simulink model "TLBO_2023"  (R2023b)
settings: Solver=ode45  StartTime=0.0  StopTime=6  MaxStep=1e-4  RelTol=1e-3  EnableMultiTasking=on
PreLoadFcn:
  | Ts_Power=1e-6;
  | Ts_Control=100e-6;
InitFcn:
  | Ts_Power=1e-6;
  | Ts_Control=100e-6;
  | Rtrans=0.142;
  | Xtrans=0.12e-6;
undefined symbols (not defined in the file): DiscIntNeverNeededParam, Ion, Lithium, sigbuilder_block
libraries: dspfdesign x80, spsSeriesRLCBranchLib x52, spsCurrentMeasurementLib x20, spsMeanLib x20, spsIdealSwitchLib x16, spsVoltageMeasurementLib x16, slpidlib x15, spsMosfetLib x14, dspindex x12, spsPWMGeneratorDCDCLib x10, spsGroundLib x10, spsBatteryLib x4
(part 4 of 4)

== system TLBO_2023/Source1/Rooftop Solar System/MPPT ==
  V_PV : Inport
  I_PV : Inport  Port=2
  Add : Sum  Inputs=+-
  Duty Cycle : Constant  Value=Dinit
  MPPT : Subsystem
  PWM Generator (DC-DC) : spsPWMGeneratorDCDCLib/PWM Generator (DC-DC)  Fsw=fc  Ts=Ts_Power
  Saturation : Saturate  UpperLimit=1  LowerLimit=0
  Scope : Scope
  Pulses : Outport  VectorParamsAs1DForOutWhenUnconnected=off
  tag scope: D=global
  wires:
  V_PV/1 -> MPPT/1(V_PV)
  I_PV/1 -> MPPT/2(I_PV)
  PWM Generator (DC-DC)/1 -> Pulses/1
  Saturation/1 -> PWM Generator (DC-DC)/1, [D]
  Add/1 -> Saturation/1, Scope/1  "D"
  MPPT/1(Delta_D) -> Add/2
  Duty Cycle/1 -> Add/1

== system TLBO_2023/Source1/Rooftop Solar System/Pmean ==
  Product : Product  RndMeth=Zero
  WkW : Gain  Gain=1/1000
  P : Outport  VectorParamsAs1DForOutWhenUnconnected=off
  V : Outport  Port=2  VectorParamsAs1DForOutWhenUnconnected=off
  wires:
  [Vmean_PV] -> Product/1, V/1
  Product/1 -> WkW/1
  [Imean_PV] -> Product/2
  WkW/1 -> P/1  "Pmean_PV (kW)"

== system TLBO_2023/Source1/Rooftop Solar System/Subsystem1 ==
  Bus Selector : BusSelector  OutputSignals=V_PV,I_PV,I_diode,Irradiance (W/m2),Temperature (deg C)
  Gain : Gain  Gain=-1
  MPPT Algorithm : Scope
  Mux2 : Mux  Inputs=2
  PV : Scope  NumInputPorts=3
  tag scope: I_PV=global, Idiode_PV=global, Ir=global, Temp=global, V_PV=global
  wires:
  [I_V_MPPT] -> Gain/1  "I_V"
  [V_PV] -> PV/1  "V_PV"
  [I_PV] -> PV/2  "I_PV"
  [Idiode_PV] -> PV/3  "Idiode_PV"
  [dI_dV_MPPT] -> Mux2/1  "dI/dV"
  Gain/1 -> Mux2/2  "-I/V"
  Mux2/1 -> MPPT Algorithm/1  "dI/dV     -I/V (magenta)"
  [m_PV] -> Bus Selector/1
  Bus Selector/1 -> [V_PV]  "<V_PV>"
  Bus Selector/2 -> [I_PV]  "<I_PV>"
  Bus Selector/4 -> [Ir]  "<Irradiance (W/m2)>"
  Bus Selector/3 -> [Idiode_PV]  "<I_diode>"
  Bus Selector/5 -> [Temp]  "<Temperature (deg C)>"

== system TLBO_2023/Source2/Rooftop Solar System/Irradiance Temp ==
  Demux : Demux  Tag=STV Demux  Outputs=2
      settings: DisplayOption=none
  FromWs : FromWorkspace  Tag=STV FromWs  VariableName=tuvar
      SigBuilderData=|
      | common.afterFinalStr = 'Extrapolate'
      | common.sampleTime = '0'
      | dataSet(1).timeRange = [0 1]
      | dataSet(1).name = 'Constant Irradiance'
      | dataSet(2).timeRange = [0 1]
      | dataSet(2).name = 'Step Irradiance'
      | dataSet(3).timeRange = [0 6]
      | dataSet(3).name = 'Ramp-up/down Irradiance'
      | sbobj.Groups(1).Name = 'Constant Irradiance'
      | sbobj.Groups(1).Signals(1).Name = 'Ir'
      | sbobj.Groups(1).Signals(1).XData = [0 1]
      | sbobj.Groups(1).Signals(1).YData = [1000 1000]
      | sbobj.Groups(1).Signals(2).Name = 'Temp'
      | sbobj.Groups(1).Signals(2).XData = [0 1 1 2]
      | sbobj.Groups(1).Signals(2).YData = [0 0 1 1]
      | sbobj.Groups(1).TimeRange = [0 1]
      | sbobj.Groups(2).Name = 'Step Irradiance'
      | sbobj.Groups(2).Signals(1).Name = 'Ir'
      | sbobj.Groups(2).Signals(1).XData = [0 0.252 0.252 1]
      | sbobj.Groups(2).Signals(1).YData = [600 600 1000 1000]
      | sbobj.Groups(2).Signals(2).Name = 'Temp'
      | sbobj.Groups(2).Signals(2).XData = [0 1 1 2]
      | sbobj.Groups(2).Signals(2).YData = [0 0 1 1]
      | sbobj.Groups(2).TimeRange = [0 1]
      | sbobj.Groups(3).Name = 'Ramp-up/down Irradiance'
      | sbobj.Groups(3).Signals(1).Name = 'Ir'
      | sbobj.Groups(3).Signals(1).XData = [0 0.6 1.1 2.2 2.7 6]
      | sbobj.Groups(3).Signals(1).YData = [1000 1000 250 250 1000 1000]
      | sbobj.Groups(3).Signals(2).Name = 'Temp'
      | sbobj.Groups(3).Signals(2).XData = [0 1.5 2.2 3 3.7 6]
      | sbobj.Groups(3).Signals(2).YData = [25 25 28 28 25 25]
      | sbobj.Groups(3).TimeRange = [0 6]
  Ir : Outport  Tag=STV Outport  VectorParamsAs1DForOutWhenUnconnected=off
  Temp : Outport  Tag=STV Outport  Port=2  VectorParamsAs1DForOutWhenUnconnected=off
  wires:
  Demux/1 -> Ir/1
  FromWs/1 -> Demux/1
  Demux/2 -> Temp/1

== system TLBO_2023/Source2/Rooftop Solar System/MPPT ==
  V_PV2 : Inport
  I_PV2 : Inport  Port=2
  Add : Sum  Inputs=+-
  Duty Cycle : Constant  Value=Dinit
  MPPT : Subsystem
  PWM Generator (DC-DC) : spsPWMGeneratorDCDCLib/PWM Generator (DC-DC)  Fsw=fc  Ts=Ts_Power
  Saturation : Saturate  UpperLimit=1  LowerLimit=0
  Scope : Scope
  Pulses : Outport  VectorParamsAs1DForOutWhenUnconnected=off
  tag scope: D2=global
  wires:
  V_PV2/1 -> MPPT/1(V_PV2)
  I_PV2/1 -> MPPT/2(I_PV2)
  PWM Generator (DC-DC)/1 -> Pulses/1
  Saturation/1 -> PWM Generator (DC-DC)/1, [D2]
  Add/1 -> Saturation/1, Scope/1  "D"
  MPPT/1(Delta_D) -> Add/2
  Duty Cycle/1 -> Add/1

== system TLBO_2023/Source2/Rooftop Solar System/Pmean ==
  Product : Product  RndMeth=Zero
  WkW : Gain  Gain=1/1000
  P : Outport  VectorParamsAs1DForOutWhenUnconnected=off
  V : Outport  Port=2  VectorParamsAs1DForOutWhenUnconnected=off
  wires:
  [Vmean_PV2] -> Product/1, V/1
  Product/1 -> WkW/1
  [Imean_PV2] -> Product/2
  WkW/1 -> P/1  "Pmean_PV (kW)"

== system TLBO_2023/Source2/Rooftop Solar System/Subsystem1 ==
  Bus Selector : BusSelector  OutputSignals=V_PV,I_PV,I_diode,Irradiance (W/m2),Temperature (deg C)
  Gain : Gain  Gain=-1
  MPPT Algorithm : Scope
  Mux2 : Mux  Inputs=2
  PV : Scope  NumInputPorts=3
  tag scope: I_PV2=global, Idiode_PV2=global, Ir2=global, Temp2=global, V_PV2=global
  wires:
  [I_V_MPPT2] -> Gain/1  "I_V"
  [V_PV2] -> PV/1  "V_PV"
  [I_PV2] -> PV/2  "I_PV"
  [Idiode_PV2] -> PV/3  "Idiode_PV"
  [dI_dV_MPPT2] -> Mux2/1  "dI/dV"
  Gain/1 -> Mux2/2  "-I/V"
  Mux2/1 -> MPPT Algorithm/1  "dI/dV     -I/V (magenta)"
  [m_PV2] -> Bus Selector/1
  Bus Selector/1 -> [V_PV2]  "<V_PV>"
  Bus Selector/2 -> [I_PV2]  "<I_PV>"
  Bus Selector/4 -> [Ir2]  "<Irradiance (W/m2)>"
  Bus Selector/3 -> [Idiode_PV2]  "<I_diode>"
  Bus Selector/5 -> [Temp2]  "<Temperature (deg C)>"

== system TLBO_2023/Source1/Rooftop Solar System/MPPT/MPPT ==
  note: Maximum power point tracking by incremental conductance method
      | --------------------------------------------------------------
      | Maximum power point is obtained when dP/dV=0  where P= V*I
      | -> d(V*I)/dV = I + V*dI/dV = 0
      | -> dI/dV = -I/V
      |
      | dI, dV  = fundamental components of I and V ripples measured with a sliding time window T_MPPT
      | I , V   = mean values of V and I measured with a sliding time window T_MPPT
      |
      | The integral regulator minimizes the error (dI/dV + I/V)
      | Regulator output = Duty cycle correction
  V_PV : Inport
  I_PV : Inport  Port=2
  Add : Sum  Inputs=+-
  Add1 : Sum
  Dead Zone : DeadZone  LowerValue=-0.05  UpperValue=0.05
  Discrete-Time Integrator : DiscreteIntegrator  SampleTime=Ts_Control  LimitOutput=on  UpperSaturationLimit=1  LowerSaturationLimit=-1  ICPrevOutput=DiscIntNeverNeededParam  ICPrevScaledInput=DiscIntNeverNeededParam
  Fourier : spsFourierLib/Fourier  Freq=1/T_MPPT  n=1  InInit=[0, 0]  Ts=Ts_Control
  Fourier1 : spsFourierLib/Fourier  Freq=1/T_MPPT  n=1  InInit=[0, 0]  Ts=Ts_Control
  MPPT Gain : Gain  Gain=5
  Mean : spsMeanLib/Mean  Freq=1/T_MPPT  Vinit=0  Ts=Ts_Control
  Mean1 : spsMeanLib/Mean  Freq=1/T_MPPT  Vinit=0  Ts=Ts_Control
  Saturation : Saturate  UpperLimit=inf  LowerLimit=eps
  Saturation1 : Saturate  UpperLimit=inf  LowerLimit=eps
  Trigonometric Function : Trigonometry  Operator=cos
  deg2rad : Gain  Gain=pi/180
  div : Product  Inputs=*/  RndMeth=Zero
  div1 : Product  Inputs=**  RndMeth=Zero
  div2 : Product  Inputs=*/  RndMeth=Zero
  Delta_D : Outport  VectorParamsAs1DForOutWhenUnconnected=off
  tag scope: I_V_MPPT=global, Imean_PV=global, Vmean_PV=global, dI_dV_MPPT=global
  wires:
  Dead Zone/1 -> MPPT Gain/1
  Saturation1/1 -> div/2
  Saturation/1 -> div2/2
  Discrete-Time Integrator/1 -> Delta_D/1
  MPPT Gain/1 -> Discrete-Time Integrator/1
  Add1/1 -> Dead Zone/1
  div2/1 -> Add1/2, [I_V_MPPT]  "I/V"
  Mean1/1 -> Saturation/1, [Vmean_PV]
  Mean/1 -> div2/1, [Imean_PV]
  div1/1 -> Add1/1, [dI_dV_MPPT]  "dI/dV"
  Trigonometric Function/1 -> div1/2
  div/1 -> div1/1
  deg2rad/1 -> Trigonometric Function/1
  Add/1 -> deg2rad/1
  Fourier1/1 -> Saturation1/1
  Fourier1/2 -> Add/2
  Fourier/2 -> Add/1
  V_PV/1 -> Mean1/1, Fourier1/1
  I_PV/1 -> Mean/1, Fourier/1
  Fourier/1 -> div/1

== system TLBO_2023/Source2/Rooftop Solar System/MPPT/MPPT ==
  note: Maximum power point tracking by incremental conductance method
      | --------------------------------------------------------------
      | Maximum power point is obtained when dP/dV=0  where P= V*I
      | -> d(V*I)/dV = I + V*dI/dV = 0
      | -> dI/dV = -I/V
      |
      | dI, dV  = fundamental components of I and V ripples measured with a sliding time window T_MPPT
      | I , V   = mean values of V and I measured with a sliding time window T_MPPT
      |
      | The integral regulator minimizes the error (dI/dV + I/V)
      | Regulator output = Duty cycle correction
  V_PV2 : Inport
  I_PV2 : Inport  Port=2
  Add : Sum  Inputs=+-
  Add1 : Sum
  Dead Zone : DeadZone  LowerValue=-0.05  UpperValue=0.05
  Discrete-Time Integrator : DiscreteIntegrator  SampleTime=Ts_Control  LimitOutput=on  UpperSaturationLimit=1  LowerSaturationLimit=-1  ICPrevOutput=DiscIntNeverNeededParam  ICPrevScaledInput=DiscIntNeverNeededParam
  Fourier : spsFourierLib/Fourier  Freq=1/T_MPPT  n=1  InInit=[0, 0]  Ts=Ts_Control
  Fourier1 : spsFourierLib/Fourier  Freq=1/T_MPPT  n=1  InInit=[0, 0]  Ts=Ts_Control
  MPPT Gain : Gain  Gain=5
  Mean : spsMeanLib/Mean  Freq=1/T_MPPT  Vinit=0  Ts=Ts_Control
  Mean1 : spsMeanLib/Mean  Freq=1/T_MPPT  Vinit=0  Ts=Ts_Control
  Saturation : Saturate  UpperLimit=inf  LowerLimit=eps
  Saturation1 : Saturate  UpperLimit=inf  LowerLimit=eps
  Trigonometric Function : Trigonometry  Operator=cos
  deg2rad : Gain  Gain=pi/180
  div : Product  Inputs=*/  RndMeth=Zero
  div1 : Product  Inputs=**  RndMeth=Zero
  div2 : Product  Inputs=*/  RndMeth=Zero
  Delta_D : Outport  VectorParamsAs1DForOutWhenUnconnected=off
  tag scope: I_V_MPPT2=global, Imean_PV2=global, Vmean_PV2=global, dI_dV_MPPT2=global
  wires:
  Dead Zone/1 -> MPPT Gain/1
  Saturation1/1 -> div/2
  Saturation/1 -> div2/2
  Discrete-Time Integrator/1 -> Delta_D/1
  MPPT Gain/1 -> Discrete-Time Integrator/1
  Add1/1 -> Dead Zone/1
  div2/1 -> Add1/2, [I_V_MPPT2]  "I/V"
  Mean1/1 -> Saturation/1, [Vmean_PV2]
  Mean/1 -> div2/1, [Imean_PV2]
  div1/1 -> Add1/1, [dI_dV_MPPT2]  "dI/dV"
  Trigonometric Function/1 -> div1/2
  div/1 -> div1/1
  deg2rad/1 -> Trigonometric Function/1
  Add/1 -> deg2rad/1
  Fourier1/1 -> Saturation1/1
  Fourier1/2 -> Add/2
  Fourier/2 -> Add/1
  V_PV2/1 -> Mean1/1, Fourier1/1
  I_PV2/1 -> Mean/1, Fourier/1
  Fourier/1 -> div/1

== matlab function TLBO_2023/Controller4/Local Controller1 ==
  data: ib_vcs input; b_control output; vbus_vcs input; c_control output; vbus_ref input; mode_vcs input; mode_sc_vcs input
function [b_control, c_control]  = fcn(ib_vcs, vbus_vcs, vbus_ref, mode_vcs, mode_sc_vcs)

% LOCAL CONTROLLER OF BATTERY-CAP SYSTEM
% 
% code to produce error signal from measured value of vbus :
% 
% (i)     Vbus > Vbus_ref +- 5% => charge battery to regulate Vbus
% (ii)    Vbus < Vbus_ref =- 5% => discharge battery to regulate Vbus
% 
% switching is controlled by signals to routers to each power switch

% v_tol = 1.05;
% vbus_max = v_tol*vbus;
% vbus_min = v_tol*vbus;

if(mode_sc_vcs==1)                      %charge state
    c_control = 1;
else                                   %discharge/standby state
    c_control = 0;
end
b_control = 1;

== matlab function TLBO_2023/Controller 2/Local Controller ==
  data: b_control output; vbus_pv2 input; vbus_ref input; mode_pv2 input
function b_control   = fcn(vbus_pv2, vbus_ref, mode_pv2)

% LOCAL CONTROLLER OF BATTERY-CAP SYSTEM
% 
% code to produce error signal from measured value of vbus :
% 
% (i)     Vbus > Vbus_ref => charge battery to regulate Vbus
% (ii)    Vbus < Vbus_ref => discharge battery to regulate Vbus
% 
% switching is controlled by signals to routers to each power switch

if(vbus_pv2>vbus_ref)                  %charge state
    b_control = 0;
else                               %discharge/standby state
    b_control = 1;
end

if(mode_pv2 == 1)
    b_control = 1;
end

== matlab function TLBO_2023/Co-operative Control1/MATLAB Function1 ==
  settings: updateMethod=DISCRETE
  data: I_ref_batt output; I_ref_sc output; mode_batt output; mode_sc output; mode_sc_pcs output; vbus_ref output; mode_sc_vcs output; V_bus input; vbus_pcs input; vbus_vcs input; PV_power input; Load_power input; SoC_batt input; SoC_sc input
function [I_ref_batt, I_ref_sc, mode_batt, mode_sc, mode_sc_pcs, vbus_ref, mode_sc_vcs] = ...
    EMS_TLBO_Simplified_Persistent(V_bus, vbus_pcs, vbus_vcs, PV_power, Load_power, SoC_batt, SoC_sc)
% EMS_TLBO_Simplified_Persistent  % TLBO-based simplified EMS with persistent variables for Simulink
%
%   This function returns fixed-size outputs for code generation and uses
%   persistent TLBO population and fitness values so the optimizer "remembers"
%   past population between Simulink steps.
%
%   Outputs (fixed size):
%       I_ref_batt   - 4x1 battery current reference [A]
%       I_ref_sc     - 2x1 supercap current reference [A]
%       mode_batt    - 4x1 battery mode flags (-1 charge, 0 idle, 1 discharge)
%       mode_sc      - 2x1 supercap mode flags (from vcs & pcs)
%       mode_sc_pcs  - scalar (pcs SC enable flag)
%       vbus_ref     - scalar nominal bus voltage (48 V)
%       mode_sc_vcs  - scalar (vcs SC enable flag)
%
%   Inputs:
%       V_bus        - vector of bus voltages (expected length >= 4)
%       vbus_pcs     - scalar: measured PCS-side bus voltage (for SC mode logic)
%       vbus_vcs     - scalar: measured VCS-side bus voltage (for SC mode logic)
%       PV_power     - vector of PV powers (per MPPT/string)
%       Load_power   - vector of load powers (per load)
%       SoC_batt     - vector length 4 (battery SoC per battery)
%       SoC_sc       - vector length 2 (supercap SoC per SC)
%
%   NOTE: This file is written to be robust: it validates sizes and clips
%   values to bounds. It also uses small eps when dividing by voltages.

% --- Fixed output sizes and defaults ---
I_ref_batt = zeros(4,1);
I_ref_sc   = zeros(2,1);
mode_batt  = zeros(4,1);
mode_sc    = zeros(2,1);
mode_sc_pcs = 0;
mode_sc_vcs = 0;
vbus_ref = 48; % Nominal DC bus voltage

% --- Constants ---
V_nom = 48;       % Nominal bus voltage
P_max_batt = 1000; % Max battery power per channel (W)
P_max_sc   = 500;  % Max supercap power per channel (W)
popSize = 15;      % TLBO population size
dim = 6;           % decision vars: [Pb1 Pb2 Pb3 Pb4 Psc1 Psc2]

% Validate inputs and expand to expected sizes when possible
if isempty(V_bus) || numel(V_bus) < 4
    % If V_bus too short, pad with nominal
    V_bus = V_nom * ones(4,1);
else
    V_bus = V_bus(:); % column
end

if isempty(PV_power), PV_power = 0; end
if isempty(Load_power), Load_power = 0; end

% Ensure SoC vectors have expected sizes (pad with mean if needed)
if isempty(SoC_batt) || numel(SoC_batt) < 4
    SoC_batt = repmat(0.5,4,1); % default 50% SoC
else
    SoC_batt = SoC_batt(:); SoC_batt = SoC_batt(1:4);
end
if isempty(SoC_sc) || numel(SoC_sc) < 2
    SoC_sc = repmat(0.5,2,1);
else
    SoC_sc = SoC_sc(:); SoC_sc = SoC_sc(1:2);
end

% --- Persistent population and fitness ---
persistent Pop Fvec initialized
if isempty(initialized) || isempty(Pop) || isempty(Fvec)
    initialized = true;
    rng('shuffle');
    % Initialize population uniformly in [-Pmax, Pmax]
    Pop = zeros(popSize, dim);
    for i = 1:popSize
        Pop(i,1:4) = -P_max_batt + 2*P_max_batt*rand(1,4); % Battery channels
        Pop(i,5:6) = -P_max_sc + 2*P_max_sc*rand(1,2);   % SC channels
    end
    % Initial fitness values
    Fvec = inf(popSize,1);
    for i = 1:popSize
        Fvec(i) = EMS_cost(Pop(i,:), V_bus, PV_power, Load_power, SoC_batt, SoC_sc, V_nom);
    end
end

% --- TLBO single iteration (teacher + learner) ---
% Teacher phase
[~, idx_best] = min(Fvec);
Xbest = Pop(idx_best,:);
meanPop = mean(Pop,1);
TF = randi([1,2]); % teaching factor 1 or 2
for i = 1:popSize
    r = rand(1,dim);
    Xnew = Pop(i,:) + r.*(Xbest - TF*meanPop);
    % Clip to bounds
    Xnew(1:4) = max(-P_max_batt, min(P_max_batt, Xnew(1:4)));
    Xnew(5:6) = max(-P_max_sc, min(P_max_sc, Xnew(5:6)));
    Jnew = EMS_cost(Xnew, V_bus, PV_power, Load_power, SoC_batt, SoC_sc, V_nom);
    if Jnew < Fvec(i)
        Pop(i,:) = Xnew; Fvec(i) = Jnew;
    end
end

% Learner phase
for i = 1:popSize
    j = randi(popSize);
    while j == i
        j = randi(popSize);
    end
    Xi = Pop(i,:); Xj = Pop(j,:);
    if Fvec(i) < Fvec(j)
        Xnew = Xi + rand(1,dim).*(Xi - Xj);
    else
        Xnew = Xi + rand(1,dim).*(Xj - Xi);
    end
    % Clip to bounds
    Xnew(1:4) = max(-P_max_batt, min(P_max_batt, Xnew(1:4)));
    Xnew(5:6) = max(-P_max_sc, min(P_max_sc, Xnew(5:6)));
    Jnew = EMS_cost(Xnew, V_bus, PV_power, Load_power, SoC_batt, SoC_sc, V_nom);
    if Jnew < Fvec(i)
        Pop(i,:) = Xnew; Fvec(i) = Jnew;
    end
end

% --- Extract best solution ---
[~, idx_best] = min(Fvec);
xbest = Pop(idx_best,:);
Pb = xbest(1:4)';   % 4x1 (W)
Psc = xbest(5:6)';   % 2x1 (W)

% --- Convert power to current references (fixed-size) ---
% Add small eps to avoid division by zero
epsV = 1e-3;
I_ref_batt(:) = Pb(:) ./ (V_bus(1:4) + epsV);
% If V_bus has >=4 entries, use elements 3 and 4 for SC nodes, otherwise use 1:2
if numel(V_bus) >= 4
    I_ref_sc(:) = Psc(:) ./ (V_bus(3:4) + epsV);
else
    I_ref_sc(:) = Psc(:) ./ (V_bus(1:2) + epsV);
end

% --- Mode flags (-1=charge, 1=discharge, 0=idle) ---
mode_batt(:) = sign(Pb(:)); mode_batt(Pb==0) = 0;
mode_sc_local = sign(Psc(:)); mode_sc_local(Psc==0) = 0;

% --- SC mode flags based on voltage thresholds ---
if nargin >= 2 && ~isempty(vbus_pcs)
    if vbus_pcs < 46
        mode_sc_pcs = 1;
    else
        mode_sc_pcs = 0;
    end
end
if nargin >= 3 && ~isempty(vbus_vcs)
    if vbus_vcs < 46
        mode_sc_vcs = 1;
    else
        mode_sc_vcs = 0;
    end
end
% Compose final mode_sc (2x1)
mode_sc = [mode_sc_local(1); mode_sc_local(2)];

end % main function

%% -----------------------------
function J = EMS_cost(P, V_bus, PV_power, Load_power, SoC_batt, SoC_sc, V_nom)
% Fitness function: minimize power mismatch + voltage deviation + usage penalties
% Inputs:
%   P - 1x6 vector: [Pb1 Pb2 Pb3 Pb4 Psc1 Psc2]

Pb = P(1:4);
Psc = P(5:6);

% Power mismatch (scalars)
P_total_storage = sum(Pb) + sum(Psc);
P_total_pv = sum(PV_power(:));
P_total_load = sum(Load_power(:));
P_err = abs(P_total_pv - P_total_load - P_total_storage);

% Voltage deviation cost (target ~V_nom)
V_bus_col = V_bus(:)';
V_err_basic = mean((V_bus_col - V_nom).^2);

% Penalty for being outside 46–50 V
lower_limit = 46; upper_limit = 50;
penalty = 0;
for k = 1:numel(V_bus_col)
    if V_bus_col(k) < lower_limit
        penalty = penalty + (lower_limit - V_bus_col(k));
    elseif V_bus_col(k) > upper_limit
        penalty = penalty + (V_bus_col(k) - upper_limit);
    end
end
V_err = V_err_basic + 5 * penalty; % add strong penalty

% SoC variance penalties (encourage balanced SoC)
SoC_err_batt = sum((SoC_batt(:) - mean(SoC_batt(:))).^2);
SoC_err_sc = sum((SoC_sc(:) - mean(SoC_sc(:))).^2);

% SC usage penalty
SC_penalty = sum(abs(Psc));

% Weighted sum (tunable weights)
w1 = 0.5; w2 = 0.7; w3 = 0.2; w4 = 0.05;
J = w1*V_err + w2*P_err + w3*(SoC_err_batt + SoC_err_sc) + w4*SC_penalty;
end

== matlab function TLBO_2023/Co-operative Control2/MATLAB Function1 ==
  settings: updateMethod=DISCRETE
  data: I_ref_batt output; I_ref_sc output; mode_batt output; mode_sc output; mode_sc_pcs output; vbus_ref output; mode_sc_vcs output; V_bus input; vbus_pcs input; vbus_vcs input; PV_power input; Load_power input; SoC_batt input; SoC_sc input
function [I_ref_batt, I_ref_sc, mode_batt, mode_sc, mode_sc_pcs, vbus_ref, mode_sc_vcs] = ...
    EMS_TLBO_Follow12(V_bus, vbus_pcs, vbus_vcs, PV_power, Load_power, SoC_batt, SoC_sc)

%% Fixed-size outputs
I_ref_batt   = zeros(4,1);   % 4x1
I_ref_sc     = zeros(2,1);   % 2x1
mode_batt    = zeros(4,1);   % 4x1
mode_sc      = zeros(2,1);   % 2x1
mode_sc_pcs  = 0;
mode_sc_vcs  = 0;
vbus_ref     = 48 * ones(4,1); % all buses targeted to 48 V

%% Parameters
V_nom        = 48;
P_max_batt   = 1000;
P_max_sc     = 500;
popSize      = 15;
dim          = 6; % [Pb1 Pb2 Pb3 Pb4 Psc3 Psc4]

lower_limit = 47;
upper_limit = 49.5;
crit_thresh = 47;
penalty_gain = 10;

w_voltage = 0.6;
w_power   = 0.8;
w_soc     = 0.2;
w_sc_use  = 0.05;

% weights for each bus (buses 3 and 4 get extra relative weight)
bus_weights = [1.0, 1.0, 1.0, 1.0];
rel_weight  = 2.0; % weight for V3~V1 and V4~V2 matching

%% Persistent TLBO state
persistent Pop Fvec initialized

if isempty(initialized)
    initialized = true;
    Pop = zeros(popSize, dim);
    for ii = 1:popSize
        Pop(ii,1:4) = -P_max_batt + 2*P_max_batt*rand(1,4);
        Pop(ii,5:6) = -P_max_sc + 2*P_max_sc*rand(1,2);
    end
    Fvec = inf(popSize,1);
    for ii=1:popSize
        Fvec(ii) = EMS_cost_follow12(Pop(ii,:), V_bus, PV_power, Load_power, SoC_batt, SoC_sc, ...
                                      V_nom, lower_limit, upper_limit, crit_thresh, bus_weights, rel_weight, penalty_gain, ...
                                      w_voltage, w_power, w_soc, w_sc_use);
    end
end

%% TLBO teacher phase
[~, idx_best] = min(Fvec);
Xbest = Pop(idx_best,:);
meanPop = mean(Pop,1);
TF = randi([1,2]);
for ii = 1:popSize
    r = rand(1,dim);
    Xnew = Pop(ii,:) + r .* ( Xbest - TF .* meanPop );
    Xnew(1:4) = max(-P_max_batt, min(P_max_batt, Xnew(1:4)));
    Xnew(5:6) = max(-P_max_sc,   min(P_max_sc,   Xnew(5:6)));
    Jnew = EMS_cost_follow12(Xnew, V_bus, PV_power, Load_power, SoC_batt, SoC_sc, ...
                              V_nom, lower_limit, upper_limit, crit_thresh, bus_weights, rel_weight, penalty_gain, ...
                              w_voltage, w_power, w_soc, w_sc_use);
    if Jnew < Fvec(ii)
        Pop(ii,:) = Xnew;
        Fvec(ii) = Jnew;
    end
end

%% TLBO learner phase
for ii = 1:popSize
    jj = randi(popSize);
    while jj == ii
        jj = randi(popSize);
    end
    Xi = Pop(ii,:); Xj = Pop(jj,:);
    if Fvec(ii) < Fvec(jj)
        Xnew = Xi + rand(1,dim) .* (Xi - Xj);
    else
        Xnew = Xi + rand(1,dim) .* (Xj - Xi);
    end
    Xnew(1:4) = max(-P_max_batt, min(P_max_batt, Xnew(1:4)));
    Xnew(5:6) = max(-P_max_sc,   min(P_max_sc,   Xnew(5:6)));
    Jnew = EMS_cost_follow12(Xnew, V_bus, PV_power, Load_power, SoC_batt, SoC_sc, ...
                              V_nom, lower_limit, upper_limit, crit_thresh, bus_weights, rel_weight, penalty_gain, ...
                              w_voltage, w_power, w_soc, w_sc_use);
    if Jnew < Fvec(ii)
        Pop(ii,:) = Xnew;
        Fvec(ii) = Jnew;
    end
end

%% Extract best solution
[~, idx_best] = min(Fvec);
xbest = Pop(idx_best,:);
Pb  = xbest(1:4);
Psc = xbest(5:6);

Pb  = max(-P_max_batt, min(P_max_batt, Pb(:)));
Psc = max(-P_max_sc,   min(P_max_sc,   Psc(:)));

% Current references
Vbus_local = V_bus(:) + 1e-6;
I_ref_batt(:) = Pb(:) ./ Vbus_local(:);
I_ref_sc(:)   = Psc(:) ./ Vbus_local(3:4);

mode_batt(:) = sign(Pb(:));
mode_batt(Pb==0) = 0;
mode_sc(:) = sign(Psc(:));
mode_sc(Psc==0) = 0;

% SC activation flags
mode_sc_pcs = double(vbus_pcs < lower_limit);
mode_sc_vcs = double(vbus_vcs < lower_limit);

end

%% --------------------------
function J = EMS_cost_follow12(P, V_bus, PV_power, Load_power, SoC_batt, SoC_sc, ...
                                V_nom, lower_limit, upper_limit, crit_thresh, bus_weights, rel_weight, penalty_gain, ...
                                w_voltage, w_power, w_soc, w_sc_use)
Pb  = P(1:4); Psc = P(5:6);
total_storage = sum(Pb) + sum(Psc);
total_PV = sum(PV_power(:));
P_err = abs(total_PV - sum(Load_power(:)) - total_storage);

% Voltage deviation from nominal
V_err_basic = sum(bus_weights(:) .* (V_bus(:) - V_nom).^2);

% Relative voltage matching: V3~V1, V4~V2
V_rel_pen = rel_weight * ((V_bus(3)-V_bus(1))^2 + (V_bus(4)-V_bus(2))^2);

% Out-of-band penalties
penalty = 0;
for k = 1:4
    vk = V_bus(k);
    if vk < lower_limit
        penalty = penalty + bus_weights(k) * (lower_limit - vk)^2;
    elseif vk > upper_limit
        penalty = penalty + bus_weights(k) * (vk - upper_limit)^2;
    end
end
if any(V_bus(:) < crit_thresh)
    idx = find(V_bus(:) < crit_thresh);
    penalty = penalty + 200 * sum((crit_thresh - V_bus(idx)).^2);
end
V_err = V_err_basic + V_rel_pen + penalty_gain*penalty;

% SoC penalties
SoC_err = sum((SoC_batt(:)-mean(SoC_batt(:))).^2) + sum((SoC_sc(:)-mean(SoC_sc(:))).^2);

% SC usage penalty
SC_penalty = sum(abs(Psc));

J = w_voltage*V_err + w_power*P_err + w_soc*SoC_err + w_sc_use*SC_penalty;
end

== matlab function TLBO_2023/Controller4/Local Controller ==
  data: b_control output; ib_vcs input; soc_b_vcs input; vbus_vcs input; vbus_ref input
function b_control   = fcn(ib_vcs, soc_b_vcs, vbus_vcs, vbus_ref)

% LOCAL CONTROLLER OF BATTERY-CAP SYSTEM
% 
% code to produce error signal from measured value of vbus :
% 
% (i)     Vbus > Vbus_ref => charge battery to regulate Vbus
% (ii)    Vbus < Vbus_ref => discharge battery to regulate Vbus
% 
% switching is controlled by signals to routers to each power switch

if(vbus_vcs>vbus_ref)                  %charge state
    b_control = 0;
else                               %discharge/standby state
    b_control = 1;
end

== matlab function TLBO_2023/Co-operative Control/MATLAB Function1 ==
  settings: updateMethod=DISCRETE
  data: V_bus input; vbus_pcs input; vbus_vcs input; PV_power input; Load_power input; SoC_batt input; SoC_sc input; I_ref_batt output; I_ref_sc output; mode_batt output; mode_sc output; mode_sc_pcs output; vbus_ref output; mode_sc_vcs output
function [I_ref_batt, I_ref_sc, mode_batt, mode_sc, mode_sc_pcs, vbus_ref, mode_sc_vcs] = ...
    EMS_TLBO_Simplified_Persistent(V_bus, vbus_pcs, vbus_vcs, PV_power, Load_power, SoC_batt, SoC_sc)
% TLBO-based simplified EMS with persistent variables for Simulink
% All outputs are fixed-size for code generation

%% Fixed output sizes
I_ref_batt = zeros(4,1);   % 4x1 battery current
I_ref_sc   = zeros(2,1);   % 2x1 supercap current
mode_batt  = zeros(4,1);   % 4x1 battery mode
mode_sc    = zeros(2,1);   % 2x1 SC mode
vbus_ref   = 48;           % Nominal DC bus voltage
mode_sc_pcs = 0;
mode_sc_vcs = 0;

%% Constants
V_nom = 48;                   % Nominal bus voltage for current calculation
P_max_batt = 100;              % Max battery power
P_max_sc   = 50;               % Max supercap power
popSize    = 15;               % TLBO population size
dim        = 6;                % [Pb1 Pb2 Pb3 Pb4 Psc3 Psc4]

%% SC mode flags based on voltage thresholds
if vbus_pcs < 46, mode_sc_pcs = 1; else mode_sc_pcs = 0; end
if vbus_vcs < 46, mode_sc_vcs = 1; else mode_sc_vcs = 0; end

%% Persistent variables
persistent Pop Fvec initialized

if isempty(initialized)
    initialized = true;
    % Initialize population uniformly in [-Pmax, Pmax]
    Pop = zeros(popSize, dim);
    for i = 1:popSize
        Pop(i,1:4) = -P_max_batt + 2*P_max_batt*rand(1,4);  % Battery
        Pop(i,5:6) = -P_max_sc + 2*P_max_sc*rand(1,2);      % SC
    end
    % Initial fitness values
    Fvec = inf(popSize,1);
    for i=1:popSize
        Fvec(i) = EMS_cost(Pop(i,:), V_bus, PV_power, Load_power, SoC_batt, SoC_sc, V_nom);
    end
end

%% TLBO single iteration (teacher + learner)
% Teacher phase
[~, idx_best] = min(Fvec);
Xbest = Pop(idx_best,:);
meanPop = mean(Pop,1);
TF = randi([1,2]);
for i=1:popSize
    r = rand(1,dim);
    Xnew = Pop(i,:) + r.*(Xbest - TF*meanPop);
    % Clip to bounds
    Xnew(1:4) = max(-P_max_batt, min(P_max_batt, Xnew(1:4)));
    Xnew(5:6) = max(-P_max_sc, min(P_max_sc, Xnew(5:6)));
    Jnew = EMS_cost(Xnew, V_bus, PV_power, Load_power, SoC_batt, SoC_sc, V_nom);
    if Jnew < Fvec(i)
        Pop(i,:) = Xnew;
        Fvec(i) = Jnew;
    end
end

% Learner phase
for i=1:popSize
    j = randi(popSize);
    while j==i, j=randi(popSize); end
    Xi = Pop(i,:); Xj = Pop(j,:);
    if Fvec(i) < Fvec(j)
        Xnew = Xi + rand(1,dim).*(Xi-Xj);
    else
        Xnew = Xi + rand(1,dim).*(Xj-Xi);
    end
    % Clip to bounds
    Xnew(1:4) = max(-P_max_batt, min(P_max_batt, Xnew(1:4)));
    Xnew(5:6) = max(-P_max_sc, min(P_max_sc, Xnew(5:6)));
    Jnew = EMS_cost(Xnew, V_bus, PV_power, Load_power, SoC_batt, SoC_sc, V_nom);
    if Jnew < Fvec(i)
        Pop(i,:) = Xnew;
        Fvec(i) = Jnew;
    end
end

%% Extract best solution
[~, idx_best] = min(Fvec);
xbest = Pop(idx_best,:);
Pb  = xbest(1:4);
Psc = xbest(5:6);

%% Convert power to current references (fixed-size)
I_ref_batt = zeros(4,1); I_ref_batt(:) = Pb(:) ./ (V_bus(:) + 1e-3);
I_ref_sc   = zeros(2,1); I_ref_sc(:)   = Psc(:) ./ (V_bus(3:4) + 1e-3);

%% Mode flags (-1=charge, 1=discharge)
mode_batt = zeros(4,1); mode_batt(:) = sign(Pb(:));
mode_batt(Pb==0)=0;
mode_sc   = zeros(2,1); mode_sc(:) = sign(Psc(:));
mode_sc(Psc==0)=0;

end

%% -----------------------------
function J = EMS_cost(P, V_bus, PV_power, Load_power, SoC_batt, SoC_sc, V_nom)
% Fitness function: minimize power mismatch + voltage deviation + usage penalties

Pb  = P(1:4);
Psc = P(5:6);

% Power mismatch
P_total_storage = sum(Pb) + sum(Psc);
P_total_pv      = sum(PV_power);
P_total_load    = sum(Load_power);
P_err = abs(P_total_pv - P_total_load - P_total_storage);

% Voltage deviation
V_err = mean((V_bus - V_nom).^2);

% SoC variance penalties
SoC_err_batt = sum((SoC_batt - mean(SoC_batt)).^2);
SoC_err_sc   = sum((SoC_sc - mean(SoC_sc)).^2);

% SC usage penalty
SC_penalty = sum(abs(Psc));

% Weighted sum
w1=1; w2=0.5; w3=0.2; w4=0.05;
J = w1*V_err + w2*P_err + w3*(SoC_err_batt + SoC_err_sc) + w4*SC_penalty;
end

== matlab function TLBO_2023/ Controller1/Local Controller ==
  data: b_control output; vbus_pv input; vbus_ref input; mode_pv input
function b_control   = fcn(vbus_pv, vbus_ref, mode_pv)

% LOCAL CONTROLLER OF BATTERY-CAP SYSTEM
% 
% code to produce error signal from measured value of vbus :
% 
% (i)     Vbus > Vbus_ref => charge battery to regulate Vbus
% (ii)    Vbus < Vbus_ref => discharge battery to regulate Vbus
% 
% switching is controlled by signals to routers to each power switch

if(vbus_pv>vbus_ref)                  %charge state
    b_control = 0;
else                               %discharge/standby state
    b_control = 1;
end

if(mode_pv == 1)
    b_control = 1;
end

== matlab function TLBO_2023/ Controller 3/Local Controller ==
  data: b_control output; ib_pcs input; soc_b_pcs input; vbus_pcs input; vbus_ref input
function b_control   = fcn(ib_pcs, soc_b_pcs, vbus_pcs, vbus_ref)

% LOCAL CONTROLLER OF BATTERY-CAP SYSTEM
% 
% code to produce error signal from measured value of vbus :
% 
% (i)     Vbus > Vbus_ref => charge battery to regulate Vbus
% (ii)    Vbus < Vbus_ref => discharge battery to regulate Vbus
% 
% switching is controlled by signals to routers to each power switch

if(vbus_pcs>vbus_ref)                  %charge state
    b_control = 0;
else                               %discharge/standby state
    b_control = 1;
end

== matlab function TLBO_2023/ Controller 3/Local Controller1 ==
  data: b_control output; ib input; vbus_pcs input; c_control output; vbus_ref input; mode_pcs input; mode_sc_pcs input
function [b_control, c_control]  = fcn(ib, vbus_pcs, vbus_ref, mode_pcs, mode_sc_pcs)

% LOCAL CONTROLLER OF BATTERY-CAP SYSTEM
% 
% code to produce error signal from measured value of vbus :
% 
% (i)     Vbus > Vbus_ref +- 5% => charge battery to regulate Vbus
% (ii)    Vbus < Vbus_ref =- 5% => discharge battery to regulate Vbus
% 
% switching is controlled by signals to routers to each power switch

% v_tol = 1.05;
% vbus_max = v_tol*vbus;
% vbus_min = v_tol*vbus;

if(mode_sc_pcs==1)                      %discharge state
    c_control = 1;
else                                   %charge/standby state
    c_control = 0;
end

b_control = 1;
